simulink model "samerHARDWARE"  (R2025b)
settings: Solver=FixedStepDiscrete  StartTime=0.0  StopTime=1500  FixedStep=0.05  RelTol=1e-3
libraries: slpidlib x6
(part 2 of 2)

== matlab function samerHARDWARE/MATLAB Function4 ==
  data: t_traj input; u_des output; shape_id output; enableFlags input
function [u_des, shape_id] = desired_trajectory_scheduler(t_traj, enableFlags)
%#codegen
% Desired trajectory scheduler for Stewart platform
%
% Inputs:
%   t_traj      : trajectory time [s]
%   enableFlags : 15x1 vector, 1 = active, 0 = inactive
%
% Outputs:
%   u_des    : [1x6] = [X Y Z Roll Pitch Yaw]
%   shape_id : active trajectory ID
%
% Units:
%   X,Y,Z in mm
%   Roll,Pitch,Yaw in rad

%% ================= BASIC SETTINGS =================
Z0 = 323.5;          % center height [mm]
Tseg = 2000;          % each active trajectory duration [s]
rampTime = 2.0;      % smooth start/end time [s]

f = 0.003;           % base frequency [Hz], period = 500 s
w = 2*pi*f;

%% ================= FORCE FLAG SIZE =================
flags = zeros(15,1);

for i = 1:15
    flags(i) = enableFlags(i);
end

%% ================= COUNT ACTIVE TRAJECTORIES =================
active_count = 0;

for i = 1:15
    if flags(i) ~= 0
        active_count = active_count + 1;
    end
end

%% ================= DEFAULT OUTPUT =================
X = 0;
Y = 0;
Z = Z0;

Roll  = 0;
Pitch = 0;
Yaw   = 0;

shape_id = 0;

u_des = zeros(1,6);
u_des(1) = X;
u_des(2) = Y;
u_des(3) = Z;
u_des(4) = Roll;
u_des(5) = Pitch;
u_des(6) = Yaw;

if active_count == 0
    return;
end

%% ================= SELECT ACTIVE TRAJECTORY =================
globalSlot = floor(t_traj / Tseg);
activeSlot = mod(globalSlot, active_count) + 1;

countNow = 0;

for i = 1:15
    if flags(i) ~= 0
        countNow = countNow + 1;

        if countNow == activeSlot
            shape_id = i;
        end
    end
end

%% ================= LOCAL TIME INSIDE SEGMENT =================
tau = t_traj - floor(t_traj / Tseg)*Tseg;

%% ================= SMOOTH GLOBAL RAMP =================
rampUp = tau / rampTime;

if rampUp > 1
    rampUp = 1;
end

if rampUp < 0
    rampUp = 0;
end

rampDown = (Tseg - tau) / rampTime;

if rampDown > 1
    rampDown = 1;
end

if rampDown < 0
    rampDown = 0;
end

% Smooth amplitude envelope.
% Keeps same path sizes, but avoids sudden jumps at segment start/end.
amp = rampUp;

if rampDown < amp
    amp = rampDown;
end

% smoothstep
amp = 1;%3*amp^2 - 2*amp^3;

%% ================= TRAJECTORIES =================

if shape_id == 1
    %% 1) EASY: X line
    Ax = 50;

    X = amp * Ax * sin(w*tau);
    Y = 0;
    Z = Z0;

elseif shape_id == 2
    %% 2) EASY: Z line
    Az = 35;

    X = 0;
    Y = 0;
    Z = Z0 + amp * Az * sin(w*tau);

elseif shape_id == 3
    %% 3) EASY: X-Z circle / ellipse
    Ax = 50;
    Az = 25;

    X = amp * Ax * sin(w*tau);
    Y = 0;
    Z = Z0 + amp * Az * cos(w*tau);

elseif shape_id == 4
    %% 4) MEDIUM: X-Z infinity
    Ax = 60;
    Az = 30;

    X = amp * Ax * sin(w*tau);
    Y = 0;
    Z = Z0 + amp * Az * sin(2*w*tau);

elseif shape_id == 5
    %% 5) MEDIUM: X-Z rectangle / square
    Ax = 60;
    Az = 30;

    Trect = 250;
    ph = tau / Trect;
    ph = ph - floor(ph);

    if ph < 0.25
        s = ph / 0.25;
        X = amp * (-Ax + 2*Ax*s);
        Z = Z0 + amp * Az;

    elseif ph < 0.50
        s = (ph - 0.25) / 0.25;
        X = amp * Ax;
        Z = Z0 + amp * (Az - 2*Az*s);

    elseif ph < 0.75
        s = (ph - 0.50) / 0.25;
        X = amp * (Ax - 2*Ax*s);
        Z = Z0 - amp * Az;

    else
        s = (ph - 0.75) / 0.25;
        X = -amp * Ax;
        Z = Z0 + amp * (-Az + 2*Az*s);
    end

    Y = 0;

elseif shape_id == 6
    %% 6) MEDIUM: X-Z triangle
    Ax = 30;
    Az = 15;

    Ttri = 30.0;
    ph = tau / Ttri;
    ph = ph - floor(ph);

    if ph < 1/3
        s = ph / (1/3);
        X = amp * (-Ax + 2*Ax*s);
        Z = Z0 - amp * Az;

    elseif ph < 2/3
        s = (ph - 1/3) / (1/3);
        X = amp * (Ax - Ax*s);
        Z = Z0 + amp * (-Az + 2*Az*s);

    else
        s = (ph - 2/3) / (1/3);
        X = amp * (0 - Ax*s);
        Z = Z0 + amp * (Az - 2*Az*s);
    end

    Y = 0;

elseif shape_id == 7
    %% 7) MEDIUM: X-Y circle with constant Z
    Ax = 25;
    Ay = 25;

    X = amp * Ax * cos(w*tau);
    Y = amp * Ay * sin(w*tau);
    Z = Z0;

elseif shape_id == 8
    %% 8) COMPLEX: 3D Lissajous
    Ax = 45;
    Ay = 24;
    Az = 24;

    X = amp * Ax * sin(w*tau);
    Y = amp * Ay * sin(2*w*tau);
    Z = Z0 + amp * Az * cos(3*w*tau);

elseif shape_id == 9
    %% 9) COMPLEX: Spiral in X-Z
    Ax = 60;
    Az = 30;

    Tspiral = Tseg;
    ph = tau / Tspiral;
    ph = ph - floor(ph);

    % Fixed reset jump:
    % old rscale = ph jumped from 1 to 0 every 60 s.
    % this keeps same max radius but returns smoothly to center.
    rscale = sin(pi*ph);

    X = amp * rscale * Ax * cos(2*w*tau);
    Y = 0;
    Z = Z0 + amp * rscale * Az * sin(2*w*tau);

elseif shape_id == 10
    %% 10) COMPLEX: 3D flower / multi-frequency curve
    f10 = 0.003;          % period = 20 s
    w10 = 2*pi*f10;

    Ax = 50;
    Ay = 40;
    Az = 25;

    flower = 1.0 + 0.15*sin(3*w10*tau);

    X = amp * Ax * flower * cos(w10*tau);
    Y = amp * Ay * flower * sin(w10*tau);
    Z = Z0 + amp * Az * sin(2*w10*tau);

    Roll  = 0;
    Pitch = 0;
    Yaw   = 0;

elseif shape_id == 11
    %% 11) COMPLEX: Circle with roll/pitch motion
    Ax = 15;
    Az = 8;

    rollAmp  = 2.0 * pi/180;
    pitchAmp = 2.0 * pi/180;

    X = amp * Ax * sin(w*tau);
    Y = 0;
    Z = Z0 + amp * Az * cos(w*tau);

    Roll  = amp * rollAmp  * sin(w*tau);
    Pitch = amp * pitchAmp * cos(w*tau);
    Yaw   = 0;

elseif shape_id == 12
    %% 12) COMPLEX: Infinity with yaw oscillation
    Ax = 15;
    Az = 8;

    yawAmp = 2.0 * pi/180;

    X = amp * Ax * sin(w*tau);
    Y = 0;
    Z = Z0 + amp * Az * sin(2*w*tau);

    Roll  = 0;
    Pitch = 0;
    Yaw   = amp * yawAmp * sin(w*tau);

elseif shape_id == 13
    %% 13) COMPLEX: Helix / corkscrew motion
    Ax = 15;
    Az = 8;

    X = amp * Ax * cos(w*tau);
    Y = amp * Ax * sin(w*tau);
    Z = Z0 + amp * Az * sin(2*w*tau);

    Roll  = 0;
    Pitch = 0;
    Yaw   = 0;

elseif shape_id == 14
    %% 14) Smooth 3D spiral / helix-like trajectory

    Tspiral = 250;
    tau14 = tau - floor(tau/Tspiral)*Tspiral;

    R = 40;       % max radius [mm]
    H = 50;       % max vertical rise [mm]
    turns = 3;    % number of turns

    s = tau14 / Tspiral;

    theta = 2*pi*turns*s;

    % Smooth envelope:
    % q starts at 0, reaches 1, then returns to 0.
    % This removes reset jump in X, Y, and Z.
    q = 0.5 * (1 - cos(2*pi*s));

    X = amp * R * q * cos(theta);
    Y = amp * R * q * sin(theta);
    Z = Z0 + amp * H * q;

    Roll  = 0;
    Pitch = 0;
    Yaw   = 0;
elseif shape_id == 15
    %% 15) 3D Tilted Square Trajectory
    Tsquare = 250;
    tau15 = tau - floor(tau/Tsquare)*Tsquare;

    side = 60;
    h = side/2;

    zTilt = 50;

    Tedge = Tsquare/4;
    edge_id = floor(tau15/Tedge);
    tau_edge = tau15 - edge_id*Tedge;

    s = tau_edge / Tedge;

    % Smooth interpolation along each edge
    s = 3*s^2 - 2*s^3;

    % 3D square corner points [X, Y, Z_offset]
    P1 = [-h, -h, -zTilt/2];
    P2 = [ h, -h,  0       ];
    P3 = [ h,  h,  zTilt/2 ];
    P4 = [-h,  h,  0       ];

    if edge_id == 0
        P_start = P1;
        P_end   = P2;

    elseif edge_id == 1
        P_start = P2;
        P_end   = P3;

    elseif edge_id == 2
        P_start = P3;
        P_end   = P4;

    else
        P_start = P4;
        P_end   = P1;
    end

    P = P_start + s * (P_end - P_start);

    X = amp * P(1);
    Y = amp * P(2);
    Z = Z0 + amp * P(3);

    Roll  = 0;
    Pitch = 0;
    Yaw   = 0;
end

%% ================= OUTPUT ROW VECTOR =================
u_des(1) = X;
u_des(2) = Y;
u_des(3) = Z;
u_des(4) = Roll;
u_des(5) = Pitch;
u_des(6) = Yaw;

end

== matlab function samerHARDWARE/Subsystem/MATLAB Function ==
  data: u input; y output; x output
function [y,x] = fcn(u)

if u >= 0
    y=1;
    x=0;
else
    y=0;
    x=1;
end

== matlab function samerHARDWARE/MATLAB Function ==
  data: u input; deltaL output
function deltaL = UPU_IK_Sim(u)
%#codegen
% UPU_IK_Sim: Inverse Kinematics for UPU Stewart Platform
%
% Input:
%   u(6x1) = [X; Y; Z; Roll; Pitch; Yaw]
%
%   X,Y,Z           -> platform center translation [mm]
%   Roll,Pitch,Yaw  -> platform rotation angles [rad]
%
% Output:
%   deltaL(6x1)     -> leg length changes from home [mm]

%% --- Force input shape ---
u = reshape(u, [6,1]);

X     = u(1);
Y     = u(2);
Z     = u(3);
Roll  = u(4);
Pitch = u(5);
Yaw   = u(6);

%% --- Geometry Definition ---
Rb = 185;   % Base radius [mm]
Rp = 150;   % Platform radius [mm]
l0 = 290;   % Nominal leg length [mm]

% Joint angle layout
angleB = deg2rad([25 49 145 169 265 289]);
angleP = deg2rad([0 74 120 194 240 314]);

b = zeros(3,6);
p = zeros(3,6);

for i = 1:6
    b(:,i) = [Rb*cos(angleB(i)); Rb*sin(angleB(i)); 0];
    p(:,i) = [Rp*cos(angleP(i)); Rp*sin(angleP(i)); 0];
end

%% --- Desired Pose ---
r = [X; Y; Z];

% Rotation matrix, ZYX order: yaw-pitch-roll
cy = cos(Yaw);   sy = sin(Yaw);
cp = cos(Pitch); sp = sin(Pitch);
cr = cos(Roll);  sr = sin(Roll);

R = [cy*cp, cy*sp*sr - sy*cr, cy*sp*cr + sy*sr;
     sy*cp, sy*sp*sr + cy*cr, sy*sp*cr - cy*sr;
     -sp,   cp*sr,            cp*cr];

%% --- Compute Leg Lengths ---
l = zeros(1,6);

for i = 1:6
    L = r + R*p(:,i) - b(:,i);
    l(i) = sqrt(L(1)^2 + L(2)^2 + L(3)^2);
end

%% --- Compute Delta Lengths ---
deltaL = l - l0;   % 6x1 column vector [mm]

end

== matlab function samerHARDWARE/Subsystem/MATLAB Function1 ==
  data: u input; y output; v input
function y = fcn(u,v)

y = u*v;

== matlab function samerHARDWARE/Subsystem/MATLAB Function2 ==
  data: u input; y output; v input
function y = fcn(u,v)

y = u*v;

== matlab function samerHARDWARE/Subsystem1/MATLAB Function ==
  data: u input; y output; x output
function [y,x] = fcn(u)

if u >= 0
    y=1;
    x=0;
else
    y=0;
    x=1;
end

== matlab function samerHARDWARE/Subsystem1/MATLAB Function1 ==
  data: u input; y output; v input
function y = fcn(u,v)

y = u*v;

== matlab function samerHARDWARE/Subsystem1/MATLAB Function2 ==
  data: u input; y output; v input
function y = fcn(u,v)

y = u*v;

== matlab function samerHARDWARE/Subsystem2/MATLAB Function ==
  data: u input; y output; x output
function [y,x] = fcn(u)

if u >= 0
    y=1;
    x=0;
else
    y=0;
    x=1;
end

== matlab function samerHARDWARE/Subsystem2/MATLAB Function1 ==
  data: u input; y output; v input
function y = fcn(u,v)

y = u*v;

== matlab function samerHARDWARE/Subsystem2/MATLAB Function2 ==
  data: u input; y output; v input
function y = fcn(u,v)

y = u*v;
